simulink model "Q3"  (R2018a)
settings: Solver=VariableStepDiscrete  StartTime=0.0  StopTime=0.5  RelTol=1e-3
undefined symbols (not defined in the file): D1, D11, Delta
libraries: powerlib x40, dspstat3 x6
settings Model: Creator=enes_  LastModifiedBy=enes_

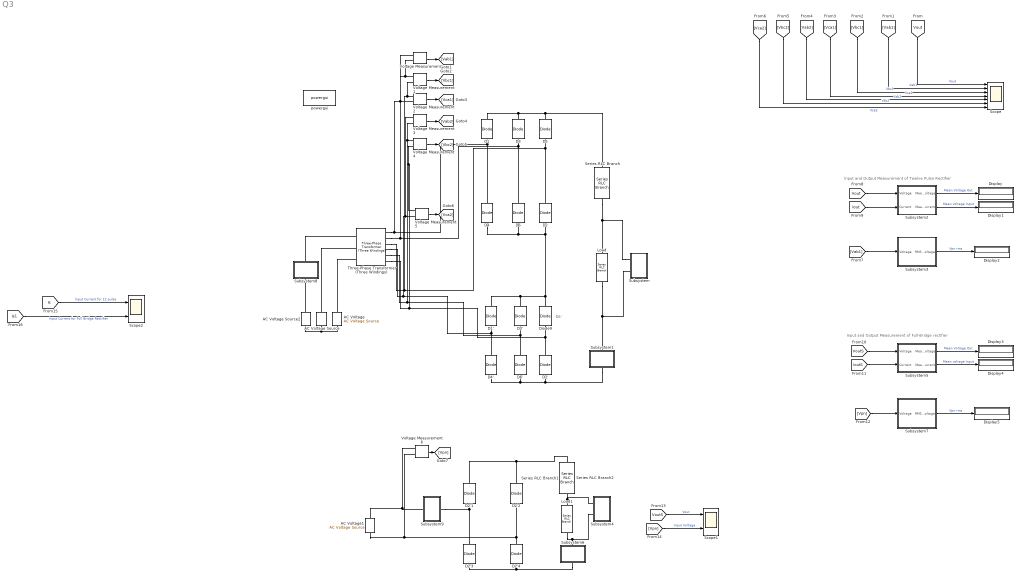
== system Q3 ==
  note: İnput and Output Measurement of Twelve Pulse Rectifier
  note: Input and Output Measurement of Full-Bridge rectifier
  note: D5'
  AC Voltage : powerlib/Electrical Sources/AC Voltage Source  Amplitude=692*sqrt(2)  Phase=-120  Frequency=50  SampleTime=0  Measurements=None  BusType=swing  Pref=10e3  Qref=0  Qmin=-inf  Qmax=+inf
  AC Voltage Source : powerlib/Electrical Sources/AC Voltage Source  Amplitude=692*sqrt(2)  Phase=120  Frequency=50  SampleTime=0  Measurements=None  BusType=swing  Pref=10e3  Qref=0  Qmin=-inf  Qmax=+inf
  AC Voltage Source2 : powerlib/Electrical Sources/AC Voltage Source  Amplitude=692*sqrt(2)  Phase=0  Frequency=50  SampleTime=0  Measurements=None  BusType=swing  Pref=10e3  Qref=0  Qmin=-inf  Qmax=+inf
  AC Voltage1 : powerlib/Electrical Sources/AC Voltage Source  Amplitude=1200*sqrt(2)  Phase=-120  Frequency=50  SampleTime=0  Measurements=None  BusType=swing  Pref=10e3  Qref=0  Qmin=-inf  Qmax=+inf
  D{1..6} (6 alike) : powerlib/Power Electronics/Diode  Ron=0.001  Lon=0  Vf=0  IC=0  UseSnubber=off  Rs=500  Cs=250e-9  Measurements=off
  D1' : powerlib/Power Electronics/Diode  Ron=0.001  Lon=0  Vf=0  IC=0  UseSnubber=off  Rs=500  Cs=250e-9  Measurements=off
  D2'{,1..4} (5 alike) : powerlib/Power Electronics/Diode  Ron=0.001  Lon=0  Vf=0  IC=0  UseSnubber=off  Rs=500  Cs=250e-9  Measurements=off
  D3' : powerlib/Power Electronics/Diode  Ron=0.001  Lon=0  Vf=0  IC=0  UseSnubber=off  Rs=500  Cs=250e-9  Measurements=off
  D4' : powerlib/Power Electronics/Diode  Ron=0.001  Lon=0  Vf=0  IC=0  UseSnubber=off  Rs=500  Cs=250e-9  Measurements=off
  D6' : powerlib/Power Electronics/Diode  Ron=0.001  Lon=0  Vf=0  IC=0  UseSnubber=off  Rs=500  Cs=250e-9  Measurements=off
  Diode9 : powerlib/Power Electronics/Diode  Ron=0.001  Lon=0  Vf=0  IC=0  UseSnubber=off  Rs=500  Cs=250e-9  Measurements=off
  Display{,1..5} (6 alike) : Display
  Load : powerlib/Elements/Series RLC Branch  LConnTagsString=__new0  RConnTagsString=__new0  BranchType=R  Resistance=10  Inductance=650e-3  SetiL0=off  InitialCurrent=0  Capacitance=1e-6  Setx0=off  InitialVoltage=0  Measurements=None
  Load1 : powerlib/Elements/Series RLC Branch  LConnTagsString=__new0  RConnTagsString=__new0  BranchType=R  Resistance=10  Inductance=650e-3  SetiL0=off  InitialCurrent=0  Capacitance=1e-6  Setx0=off  InitialVoltage=0  Measurements=None
  Scope : Scope  NumInputPorts=7
  Scope1 : Scope  NumInputPorts=2
  Scope2 : Scope  NumInputPorts=2
  Series RLC Branch : powerlib/Elements/Series RLC Branch  LConnTagsString=__new0  RConnTagsString=__new0  BranchType=L  Resistance=1  Inductance=1  SetiL0=off  InitialCurrent=0  Capacitance=1e-6  Setx0=off  InitialVoltage=0  Measurements=None
  Series RLC Branch1 : powerlib/Elements/Series RLC Branch  LConnTagsString=__new0  RConnTagsString=__new0  BranchType=L  Resistance=1  Inductance=1  SetiL0=off  InitialCurrent=0  Capacitance=1e-6  Setx0=off  InitialVoltage=0  Measurements=None
  Series RLC Branch2 : powerlib/Elements/Series RLC Branch  LConnTagsString=__new0  RConnTagsString=__new0  BranchType=L  Resistance=1  Inductance=1  SetiL0=off  InitialCurrent=0  Capacitance=1e-6  Setx0=off  InitialVoltage=0  Measurements=None
  Subsystem : Subsystem
  Subsystem1 : Subsystem
  Subsystem2 : Subsystem
  Subsystem3 : Subsystem
  Subsystem4 : Subsystem
  Subsystem5 : Subsystem
  Subsystem6 : Subsystem
  Subsystem7 : Subsystem
  Subsystem8 : Subsystem
  Subsystem9 : Subsystem
  Three-Phase Transformer (Three Windings) : powerlib/Elements/Three-Phase Transformer (Three Windings)  Winding1Connection=Delta (D1)  Winding2Connection=Y  Winding3Connection=Delta (D11)  CoreType=Three single-phase transformers  SetSaturation=off  Hysteresis=off  DataFile='hysteresis'  SetInitialFlux=off  Measurements=None  UNITS=pu  NominalPower=[ 250e3 , 50 ]  Winding1=[ 300 , 0.002 , 0.08 ]  Winding2=[ 100 , 0.002 , 0.08 ]  Winding3=[ 100 , 0.002 , 0.08 ]  Rm=500  Lm=500  L0=0.5  Saturation=[ 0,0 ; 0.0024,1.2 ; 1.0,1.52 ]  InitialFluxes=[0.8 -0.8 0.7]  MoreParameters=off  BreakLoop=off  DataType=off  TransfoNumber=1
      settings: SourceProductName=Simscape Power Systems  SourceProductBaseCode=PS
  Voltage Measurement{,1..6} (7 alike) : powerlib/Measurements/Voltage Measurement  PhasorSimulation=off  OutputType=Complex  PSBequivalent=0
  powergui : powerlib/powergui  Priority=1  SimulationMode=Discrete  SampleTime=1e-6  frequency=60  Iterations=50  frequencyindice=50  Pbase=100e6  ErrMax=1e-4  UnitsV=kV  UnitsW=MW  buscounter=0  FunctionMessages=off  echomessages=off  EnableUseOfTLC=off  CurrentSourceSwitches=off  DisableSnubberDevices=off  DisableRonSwitches=off  DisableVfSwitches=off  DisplayEquations=off  SolverType=Tustin/Backward Euler (TBE)  Interpol=off  ExternalGateDelay=off  methode=off  Ts=100  x0status=blocks  SPID=on  SwTol=0  HookPort=off  RestoreLinks=warning  ResistiveCurrentMeasurement=off  Frange=[0:2:500]  Ylog=off  Xlog=on  ShowGrid=off  save=off  variable=ZData  structure=0  ZoomFFT=off  StartTime=0.0  cycles=1  DisplayStyle=1  fundamental=60  FreqAxis=off  MaxFrequency=1000  frequencyindicesteady=1  RmsSteady=1  display=off
  wires:
  [Vout] -> Scope/1  "Vout"
  Voltage Measurement/1 -> [Vab1]
  Voltage Measurement1/1 -> [Vbc1]
  Voltage Measurement2/1 -> [Vca1]
  Voltage Measurement3/1 -> [Vab2]
  Voltage Measurement4/1 -> [Vbc2]
  Voltage Measurement5/1 -> [Vca2]
  [Vab1] -> Scope/2  "Vab1"
  [Vbc1] -> Scope/3  "Vbc1"
  [Vca1] -> Scope/4  "Vca1"
  [Vab2] -> Scope/5  "Vab2"
  [Vbc2] -> Scope/6  "Vbc2"
  [Vca2] -> Scope/7  "Vca2"
  Voltage Measurement6/1 -> [Vpn]
  Subsystem5/1(Mean Voltage) -> Display3/1  "Mean Voltage Out"
  Subsystem5/2(Mean Current) -> Display4/1  "Mean voltage Input"
  [VoutS] -> Subsystem5/1(Voltage)
  [IoutS] -> Subsystem5/2(Current)
  Subsystem7/1(RMS voltage) -> Display5/1  "Vpn rms"
  [Vpn] -> Subsystem7/1(Voltage)
  Subsystem2/1(Mean Voltage) -> Display/1  "Mean Voltage Out"
  Subsystem2/2(Mean Current) -> Display1/1  "Mean voltage Input"
  [Iout] -> Subsystem2/2(Current)
  Subsystem3/1(RMS voltage) -> Display2/1  "Vpn rms"
  [Vout] -> Subsystem2/1(Voltage)
  [Vab1] -> Subsystem3/1(Voltage)
  [VoutS] -> Scope1/1  "Vout"
  [Vpn] -> Scope1/2  "Input Voltage"
  [Is] -> Scope2/1  "İnput Current for 12 pulse"
  [Is1] -> Scope2/2  "Input Current for Full Bridge Rectifier"
  connections:
  D2/LConn1 -- D3'/RConn1 -- D1'/RConn1 -- Diode9/RConn1 -- D6/LConn1 -- D4/LConn1
  Three-Phase Transformer (Three Windings)/RConn6 -- Voltage Measurement4/LConn2 -- Voltage Measurement5/LConn1 -- D2'/RConn1 -- Diode9/LConn1
  Three-Phase Transformer (Three Windings)/RConn2 -- Voltage Measurement/LConn2 -- Voltage Measurement1/LConn1 -- D3/LConn1 -- D6/RConn1
  D3'/LConn1 -- Three-Phase Transformer (Three Windings)/RConn5 -- Voltage Measurement3/LConn2 -- Voltage Measurement4/LConn1 -- D6'/RConn1
  D1/LConn1 -- Voltage Measurement2/LConn2 -- Voltage Measurement/LConn1 -- Three-Phase Transformer (Three Windings)/RConn1 -- D4/RConn1
  Subsystem/LConn1 -- Series RLC Branch/RConn1 -- Load/LConn1
  Three-Phase Transformer (Three Windings)/RConn4 -- Voltage Measurement3/LConn1 -- Voltage Measurement5/LConn2 -- D1'/LConn1 -- D4'/RConn1
  AC Voltage Source/RConn1 -- Three-Phase Transformer (Three Windings)/LConn2
  AC Voltage Source2/RConn1 -- Subsystem8/LConn1
  AC Voltage/RConn1 -- Three-Phase Transformer (Three Windings)/LConn3
  AC Voltage Source2/LConn1 -- AC Voltage/LConn1 -- AC Voltage Source/LConn1
  D4'/LConn1 -- D6'/LConn1 -- Subsystem1/RConn1 -- D2'/LConn1
  Load/RConn1 -- Subsystem/LConn2 -- Subsystem1/LConn1
  Subsystem4/LConn1 -- Load1/LConn1 -- Series RLC Branch1/RConn1
  D2'1/LConn1 -- Subsystem9/RConn1 -- D2'3/RConn1
  Load1/RConn1 -- Subsystem4/LConn2 -- Subsystem6/LConn1
  D2'4/RConn1 -- D2'2/LConn1 -- AC Voltage1/LConn1 -- Voltage Measurement6/LConn2
  Subsystem6/RConn1 -- D2'3/LConn1 -- D2'4/LConn1
  D2/RConn1 -- Three-Phase Transformer (Three Windings)/RConn3 -- Voltage Measurement1/LConn2 -- Voltage Measurement2/LConn1 -- D5/LConn1
  Subsystem8/RConn1 -- Three-Phase Transformer (Three Windings)/LConn1
  AC Voltage1/RConn1 -- Subsystem9/LConn1 -- Voltage Measurement6/LConn1
  D1/RConn1 -- D3/RConn1 -- Series RLC Branch/LConn1 -- D5/RConn1
  Series RLC Branch1/LConn1 -- D2'1/RConn1 -- D2'2/RConn1

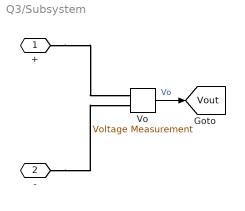
== system Q3/Subsystem ==
  Vo : powerlib/Measurements/Voltage Measurement  PhasorSimulation=off  OutputType=Complex  PSBequivalent=0
  + : PMIOPort  Side=Left
  - : PMIOPort  Port=2  Side=Left
  tag scope: Vout=global
  wires:
  Vo/1 -> [Vout]  "Vo"
  connections:
  -/RConn1 -- Vo/LConn2
  +/RConn1 -- Vo/LConn1

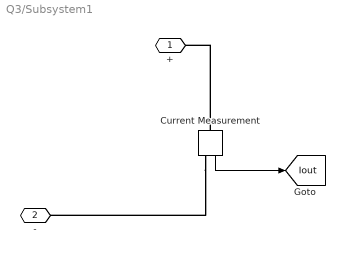
== system Q3/Subsystem1 ==
  Current Measurement : powerlib/Measurements/Current Measurement  PhasorSimulation=off  OutputType=Complex  PSBequivalent=0
  + : PMIOPort  Side=Left
  - : PMIOPort  Port=2  Side=Right
  tag scope: Iout=global
  wires:
  Current Measurement/1 -> [Iout]
  connections:
  Current Measurement/LConn1 -- +/RConn1
  Current Measurement/RConn1 -- -/RConn1

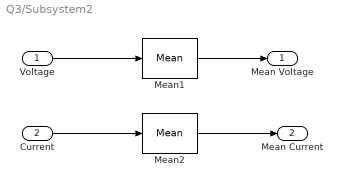
== system Q3/Subsystem2 ==
  Voltage : Inport
  Current : Inport  Port=2
  Mean1 : dspstat3/Mean  run=on  InputProcessing=Columns as channels (frame based)  reset_popup=None  directionMode=Each column  dimension=1  roiEnable=off  roiType=Rectangles  roiPortion=Entire ROI  roiOutput=Individual statistics for each ROI  roiFlag=off  roundingMode=Floor  overflowMode=off  outputDataTypeStr=Inherit: Same as accumulator  outputMin=[]  outputMax=[]  outputLastDataTypeStr=Inherit: Same as accumulator
  Mean2 : dspstat3/Mean  run=on  InputProcessing=Columns as channels (frame based)  reset_popup=None  directionMode=Each column  dimension=1  roiEnable=off  roiType=Rectangles  roiPortion=Entire ROI  roiOutput=Individual statistics for each ROI  roiFlag=off  roundingMode=Floor  overflowMode=off  outputDataTypeStr=Inherit: Same as accumulator  outputMin=[]  outputMax=[]  outputLastDataTypeStr=Inherit: Same as accumulator
  Mean Voltage : Outport
  Mean Current : Outport  Port=2
  wires:
  Mean2/1 -> Mean Current/1
  Voltage/1 -> Mean1/1
  Mean1/1 -> Mean Voltage/1
  Current/1 -> Mean2/1

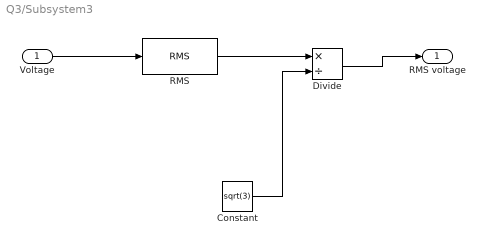
== system Q3/Subsystem3 ==
  Voltage : Inport
  Constant : Constant  Value=sqrt(3)
  Divide : Product  Inputs=*/
  RMS : dspstat3/RMS  run=on  directionMode=Each column  dimension=1  InputProcessing=Columns as channels (frame based)  reset_popup=None
  RMS voltage : Outport
  wires:
  Voltage/1 -> RMS/1
  RMS/1 -> Divide/1
  Divide/1 -> RMS voltage/1
  Constant/1 -> Divide/2

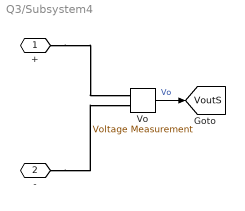
== system Q3/Subsystem4 ==
  Vo : powerlib/Measurements/Voltage Measurement  PhasorSimulation=off  OutputType=Complex  PSBequivalent=0
  + : PMIOPort  Side=Left
  - : PMIOPort  Port=2  Side=Left
  tag scope: VoutS=global
  wires:
  Vo/1 -> [VoutS]  "Vo"
  connections:
  -/RConn1 -- Vo/LConn2
  +/RConn1 -- Vo/LConn1

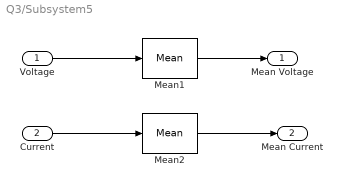
== system Q3/Subsystem5 ==
  Voltage : Inport
  Current : Inport  Port=2
  Mean1 : dspstat3/Mean  run=on  InputProcessing=Columns as channels (frame based)  reset_popup=None  directionMode=Each column  dimension=1  roiEnable=off  roiType=Rectangles  roiPortion=Entire ROI  roiOutput=Individual statistics for each ROI  roiFlag=off  roundingMode=Floor  overflowMode=off  outputDataTypeStr=Inherit: Same as accumulator  outputMin=[]  outputMax=[]  outputLastDataTypeStr=Inherit: Same as accumulator
  Mean2 : dspstat3/Mean  run=on  InputProcessing=Columns as channels (frame based)  reset_popup=None  directionMode=Each column  dimension=1  roiEnable=off  roiType=Rectangles  roiPortion=Entire ROI  roiOutput=Individual statistics for each ROI  roiFlag=off  roundingMode=Floor  overflowMode=off  outputDataTypeStr=Inherit: Same as accumulator  outputMin=[]  outputMax=[]  outputLastDataTypeStr=Inherit: Same as accumulator
  Mean Voltage : Outport
  Mean Current : Outport  Port=2
  wires:
  Mean2/1 -> Mean Current/1
  Voltage/1 -> Mean1/1
  Mean1/1 -> Mean Voltage/1
  Current/1 -> Mean2/1

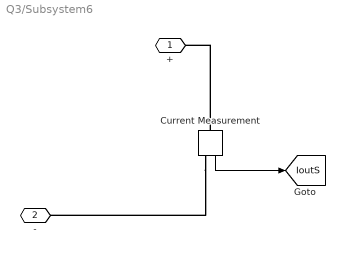
== system Q3/Subsystem6 ==
  Current Measurement : powerlib/Measurements/Current Measurement  PhasorSimulation=off  OutputType=Complex  PSBequivalent=0
  + : PMIOPort  Side=Left
  - : PMIOPort  Port=2  Side=Right
  tag scope: IoutS=global
  wires:
  Current Measurement/1 -> [IoutS]
  connections:
  Current Measurement/LConn1 -- +/RConn1
  Current Measurement/RConn1 -- -/RConn1

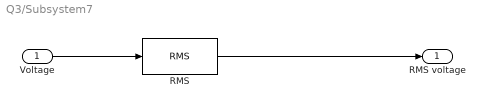
== system Q3/Subsystem7 ==
  Voltage : Inport
  RMS : dspstat3/RMS  run=on  directionMode=Each column  dimension=1  InputProcessing=Columns as channels (frame based)  reset_popup=None
  RMS voltage : Outport
  wires:
  Voltage/1 -> RMS/1
  RMS/1 -> RMS voltage/1

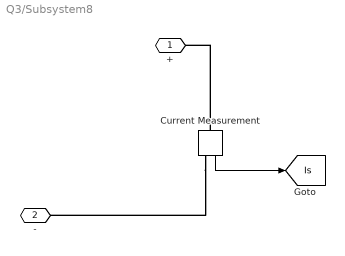
== system Q3/Subsystem8 ==
  Current Measurement : powerlib/Measurements/Current Measurement  PhasorSimulation=off  OutputType=Complex  PSBequivalent=0
  + : PMIOPort  Side=Left
  - : PMIOPort  Port=2  Side=Right
  tag scope: Is=global
  wires:
  Current Measurement/1 -> [Is]
  connections:
  Current Measurement/LConn1 -- +/RConn1
  Current Measurement/RConn1 -- -/RConn1

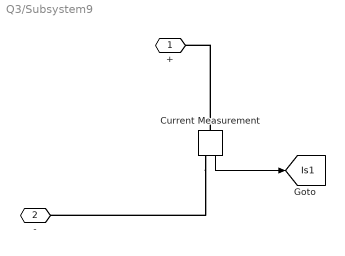
== system Q3/Subsystem9 ==
  Current Measurement : powerlib/Measurements/Current Measurement  PhasorSimulation=off  OutputType=Complex  PSBequivalent=0
  + : PMIOPort  Side=Left
  - : PMIOPort  Port=2  Side=Right
  tag scope: Is1=global
  wires:
  Current Measurement/1 -> [Is1]
  connections:
  Current Measurement/LConn1 -- +/RConn1
  Current Measurement/RConn1 -- -/RConn1
